simulink model "ev_pilot_handshake"  (R2024b)
settings: Solver=FixedStepAuto  StartTime=0.0  StopTime=5  FixedStep=1e-6  RelTol=1e-3
libraries: fl_lib x23, nesl_utility x13, ee_lib x2, simulink x1
settings Model: Creator=Shakeb  LastModifiedBy=Shakeb

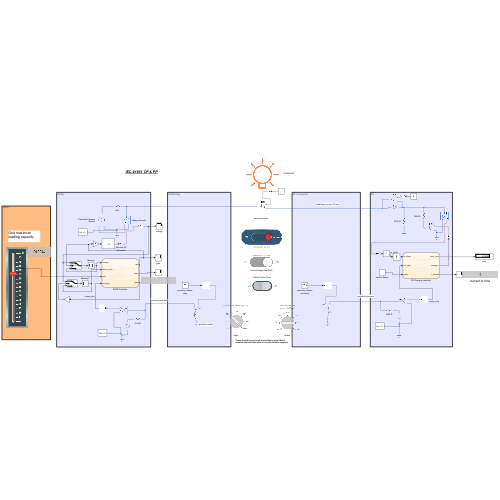
[thumbnail: Simulink's stored preview of the top-level diagram]
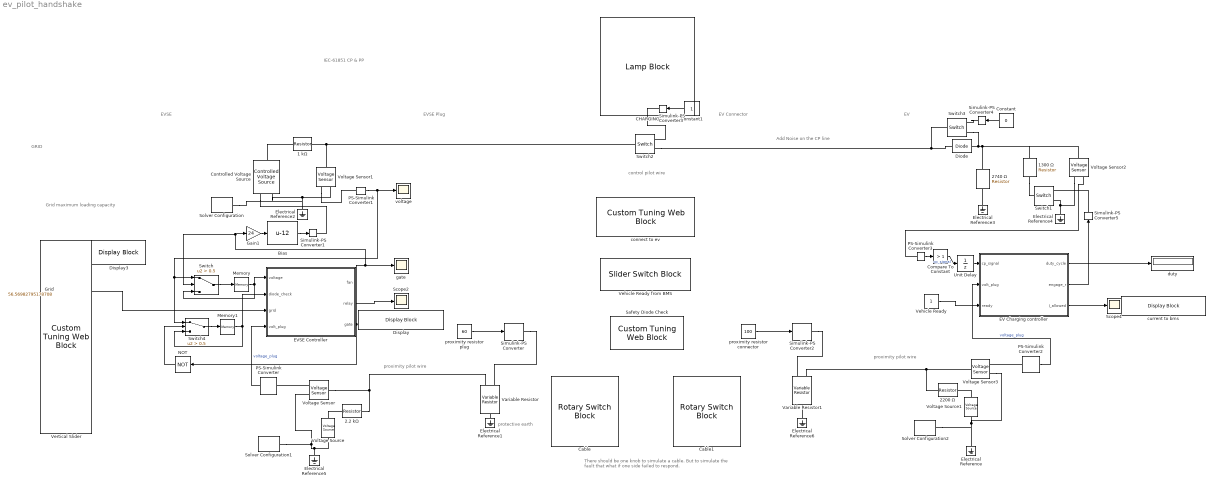
== system ev_pilot_handshake ==
  note: Grid maximum loading capacity
  note: GRID
  note: Add Noise on the CP line
  note: IEC-61851 CP & PP
  note: There should be one knob to simulate a cable. But to simulate the fault that what if one side failed to respond.
  note: protective earth
  note: control pilot wire
  note: proximity pilot wire
  note: EV
  note: EV Connector
  note: EVSE Plug
  note: EVSE
  note: proximity pilot wire
  1 kΩ : fl_lib/Electrical/Electrical Elements/Resistor  R=1000 Ohm  i_specify=off  i_priority=None  i=0 A  i_nominal_specify=off  i_nominal_value=1  i_nominal_unit=A  v_specify=off  v_priority=None  v=0 V  v_nominal_specify=off  v_nominal_value=1  v_nominal_unit=V
  1300 Ω : fl_lib/Electrical/Electrical Elements/Resistor  R=1300 Ohm  i_specify=off  i_priority=None  i=0 A  i_nominal_specify=off  i_nominal_value=1  i_nominal_unit=A  v_specify=off  v_priority=None  v=0 V  v_nominal_specify=off  v_nominal_value=1  v_nominal_unit=V
  2.2 kΩ : fl_lib/Electrical/Electrical Elements/Resistor  R=2200 Ohm  i_specify=off  i_priority=None  i=0 A  i_nominal_specify=off  i_nominal_value=1  i_nominal_unit=A  v_specify=off  v_priority=None  v=0 V  v_nominal_specify=off  v_nominal_value=1  v_nominal_unit=V
  2200 Ω : fl_lib/Electrical/Electrical Elements/Resistor  R=2200 Ohm  i_specify=off  i_priority=None  i=0 A  i_nominal_specify=off  i_nominal_value=1  i_nominal_unit=A  v_specify=off  v_priority=None  v=0 V  v_nominal_specify=off  v_nominal_value=1  v_nominal_unit=V
  2740 Ω : fl_lib/Electrical/Electrical Elements/Resistor  R=2740 Ohm  i_specify=off  i_priority=None  i=0 A  i_nominal_specify=off  i_nominal_value=1  i_nominal_unit=A  v_specify=off  v_priority=None  v=0 V  v_nominal_specify=off  v_nominal_value=1  v_nominal_unit=V
  Bias : Bias  Bias=-12  SaturateOnIntegerOverflow=off
  CHARGING : LampBlock  LabelPosition=Hide  Icon=LightingSwitch
  Cable : RotarySwitchBlock
      settings: Values={{'fault', '13A', '16A', '20A', '32A', '63A', 'short'}, [4500 1500 1000 680 220 100 60]}
  Cable1 : RotarySwitchBlock
      settings: Values={{'fault', '13A', '16A', '20A', '32A', '63A', 'short'}, [4500 1500 1000 680 220 100 60]}
  Compare To Constant : simulink/Logic and Bit Operations/Compare To Constant  relop=>  const=1  OutDataTypeStr=boolean
  Constant : Constant  Value=0
  Constant1 : Constant
  Controlled Voltage Source : fl_lib/Electrical/Electrical Sources/Controlled Voltage Source
  Diode : fl_lib/Electrical/Electrical Elements/Diode  Vf=0.6 V  Ron=0.3 Ohm  Goff=1e-8 1/Ohm  i_specify=off  i_priority=None  i=0 A  i_nominal_specify=off  i_nominal_value=1  i_nominal_unit=A  v_specify=off  v_priority=None  v=0 V  v_nominal_specify=off  v_nominal_value=1  v_nominal_unit=V
  Display : DisplayBlock  LabelPosition=Hide  Transparency=1
  Display3 : DisplayBlock  LabelPosition=Hide  Transparency=1
  EV Charging controller : Stateflow chart  TreatAsAtomicUnit=on
  EVSE Controller : Stateflow chart  TreatAsAtomicUnit=on
  Electrical Reference{,1..6} (7 alike) : fl_lib/Electrical/Electrical Elements/Electrical Reference
  Gain1 : Gain  Gain=24
  Grid : Constant  Value=56.56982795178708
  Memory : Memory  InitialCondition=12  InheritSampleTime=on
  Memory1 : Memory  InitialCondition=-12  InheritSampleTime=on
  NOT : Logic  Operator=NOT  IconShape=distinctive  AllPortsSameDT=off  OutDataTypeStr=boolean
  PS-Simulink Converter{,1..3} (4 alike) : nesl_utility/PS-Simulink Converter  PhysicalDomain=network_engine_domain  SubClassName=ps_output  LeftPortType=input  RightPortType=output  PseudoPeriodic=off  Frequencies=[]  VectorFormat=inherit  Unit=inherit  AffineConversion=off
  Safety Diode Check : CustomTuningWebBlock  LabelPosition=Hide  ShowInitialText=on  Configuration="{\"components\":[{\"name\":\"CustomSwitchStateComponent\",\"settings\":{\"position\":[0,0,1,1],\"states\":[{\"HitRegion\":{\"position\":[0,0,0.5,1]},\"Image\":{\"position\":[0.13,0,1,0.75],\"size\":[1,0.75],\"src\":\"data:image\\/svg+xml;base64,PHN2ZyB4bWxucz0iaHR0cDovL3d3dy53My5vcmcvMjAwMC9zdmciIHhtbG5zOnhsaW5rPSJodHRwOi8vd3d3LnczLm9yZy8xOTk5L3hsaW5rIiB2aWV3Qm94PSIwIDAgNzUgMjQuOCI+PGRlZnM+PHN0eWxlPi5jbHMtMXtmaWxsOnVybCgjcmFkaWFsLWdyYWRpZW50KTt9LmNscy0ye2ZpbGw6dXJsKCNyYWRpYWwtZ3JhZGllbnQtMik7fS5jbHMtM3tzdHJva2U6I2IyMDAwMDtzdHJva2Utd2lkdGg6MC4yNXB4O2ZpbGw6dXJsKCNsaW5lYXItZ3JhZGllbnQpO30uY2xzLTR7ZmlsbDp1cmwoI2xpbmVhci1ncmFkaWVudC0yKTt9LmNs ...(+3576 chars)\",\"srcOrientation\":\"Right\"},\"Label\":{\"color\":[0.5019607843137255,0.5019607843137255,0.5019607843137255],\"icon\":{\"size\":[0,0],\"src\":[],\"srcOrientation\":\"Right\"},\"iconOffset\":0,\"iconPlacement\":\"left\",\"opacity\":1,\"position\":[0.5,0.08],\"show\":true,\"text\":{\"content\":\"On\",\"font\":\"Helvetica\"}},\"Value\":0},{\"HitRegion\":{\"position\":[0,0.5,0.5,1]},\"Image\":{\"position\":[0.13,0,1,0.75],\"size\":[1,0.75],\"src\":\"data:image\\/svg+xml;base64,PHN2ZyB4bWxucz0iaHR0cDovL3d3dy53My5vcmcvMjAwMC9zdmciIHhtbG5zOnhsaW5rPSJodHRwOi8vd3d3LnczLm9yZy8xOTk5L3hsaW5rIiB2aWV3Qm94PSIwIDAgNzUgMjQuOCI+PGRlZnM+PHN0eWxlPi5jbHMtMXtmaWxsOnVybCgjcmFkaWFsLWdyYWRpZW50KTt9LmNscy0ye2ZpbGw6dXJsKCNyYWRpYWwtZ3JhZGllbnQtMik7fS5jbHMtM3tzdHJva2U6I2IyMDAwMDtzdHJva2Utd2lkdGg6MC4yNXB4O2ZpbGw6dXJsKCNsaW5lYXItZ3JhZGllbnQpO30uY2xzLTR7ZmlsbDp1cmwoI2xpbmVhci1ncmFkaWVudC0yKTt9LmNs ...(+3520 chars)\",\"srcOrientation\":\"Right\"},\"Label\":{\"color\":[0.5019607843137255,0.5019607843137255,0.5019607843137255],\"icon\":{\"size\":[0,0],\"src\":[],\"srcOrientation\":\"Right\"},\"iconOffset\":0,\"iconPlacement\":\"left\",\"opacity\":1,\"position\":[0.5,0.92],\"show\":true,\"text\":{\"content\":\"Off\",\"font\":\"Helvetica\"}},\"Value\":1}]}},{\"name\":\"BackgroundImageComponent\",\"settings\":{\"image\":{\"size\":[155,70],\"src\":\"default\",\"srcOrientation\":\"Right\"},\"position\":[0,0,1,1],\"scaleMode\":\"0\"}},{\"name\":\"ForegroundImageComponent\",\"settings\":{\"image\":{\"size\":[0,0],\"src\":\"default\",\"srcOrientation\":[]},\"isForeground\":1,\"position\":[0,0,1,1],\"scaleMode\":\"0\"}}],\"settings\":{\"BindingType\":\"param\",\"backgroundColor\":[0,0,255,\"1\"],\"backgroundOffset\":0.14,\"fixedAspectRatio\":\"on\",\"foregroundColor\":[234,234,234],\"showBackgroundColor\":false,\"variant\":\"rocker\",\"version\":\"R2024b\"},\"type\":\"Switch\"}"  CustomBackgroundColor="{\"color\":[1,1,1],\"show\":true}"
  Scope2 : Scope
  Scope4 : Scope
  Simulink-PS Converter{,1..5} (6 alike) : nesl_utility/Simulink-PS Converter  PhysicalDomain=network_engine_domain  SubClassName=ps_input  LeftPortType=input  RightPortType=output  PseudoPeriodic=off  Frequencies=[]  NoiseDistribution=none  NoiseParameters=[]  Unit=1  AffineConversion=off  FilteringAndDerivatives=provide  SimscapeFilterOrder=1  InputFilterTimeConstant=0.001  UdotUserProvided=0
  Solver Configuration : nesl_utility/Solver Configuration  PhysicalDomain=network_engine_domain  SubClassName=solver  LeftPortType=input  RightPortType=generic  Tones=[]  Harmonics=[]  SimulateNoise=off  Profile=off  UseLocalSampling=off  EnableSwitchedLinearOptims=on  FrequencyDomain=off  UseCCode=off  RelTol=0.001  AbsTol=0.001  MinStep=1e-09  ToWorkspace=off  RevertToSquareIcSolve=off  NumHomotopyIterations=100  PhasorMode=off  PhasorModeNumHarmonics=1  ConsistencySolver=NEWTON_XTOL_AFTER_FTOL  IndexReductionMethod=DerivativeReplacement  DoDC=off  ResidualTolerance=1e-09  ConsistencyTolSource=GLOBAL  ConsistencyAbsTol=0.001  ConsistencyRelTol=0.001  ConsistencyTolFactor=0.001  UseLocalSolver=off  LocalSolverChoice=NE_BACKWARD_EULER_ADVANCER  ResolveIndetEquations=on  FunctionEvalNumThread=1  LocalSolverSampleTime=0.001  DoFixedCost=off  MaxNonlinIter=3  MaxModeIter=2  ComputeImpulses=off  ImpulseIterations=2  LinearAlgebra=auto  LinearAlgebraNumThread=0  EquationFormulation=NE_TIME_EF  DelaysMemoryBudget=1024  AutomaticFiltering=on  FilteringTimeConstant=0.001  PartitionStorageMethod=AS_NEEDED  PartitionMemoryBudget=1024  PartitionMethod=ROBUST  MultibodyUseLocalSolver=off  MultibodyLocalSolverChoice=ODE1  MultibodyLocalSolverSampleTime=0.001
  Solver Configuration1 : nesl_utility/Solver Configuration  PhysicalDomain=network_engine_domain  SubClassName=solver  LeftPortType=input  RightPortType=generic  Tones=[]  Harmonics=[]  SimulateNoise=off  Profile=off  UseLocalSampling=off  EnableSwitchedLinearOptims=on  FrequencyDomain=off  UseCCode=off  RelTol=0.001  AbsTol=0.001  MinStep=1e-09  ToWorkspace=off  RevertToSquareIcSolve=off  NumHomotopyIterations=100  PhasorMode=off  PhasorModeNumHarmonics=1  ConsistencySolver=NEWTON_XTOL_AFTER_FTOL  IndexReductionMethod=DerivativeReplacement  DoDC=off  ResidualTolerance=1e-09  ConsistencyTolSource=GLOBAL  ConsistencyAbsTol=0.001  ConsistencyRelTol=0.001  ConsistencyTolFactor=0.001  UseLocalSolver=off  LocalSolverChoice=NE_BACKWARD_EULER_ADVANCER  ResolveIndetEquations=on  FunctionEvalNumThread=1  LocalSolverSampleTime=0.001  DoFixedCost=off  MaxNonlinIter=3  MaxModeIter=2  ComputeImpulses=off  ImpulseIterations=2  LinearAlgebra=auto  LinearAlgebraNumThread=0  EquationFormulation=NE_TIME_EF  DelaysMemoryBudget=1024  AutomaticFiltering=on  FilteringTimeConstant=0.001  PartitionStorageMethod=AS_NEEDED  PartitionMemoryBudget=1024  PartitionMethod=ROBUST  MultibodyUseLocalSolver=off  MultibodyLocalSolverChoice=ODE1  MultibodyLocalSolverSampleTime=0.001
  Solver Configuration2 : nesl_utility/Solver Configuration  PhysicalDomain=network_engine_domain  SubClassName=solver  LeftPortType=input  RightPortType=generic  Tones=[]  Harmonics=[]  SimulateNoise=off  Profile=off  UseLocalSampling=off  EnableSwitchedLinearOptims=on  FrequencyDomain=off  UseCCode=off  RelTol=0.001  AbsTol=0.001  MinStep=1e-09  ToWorkspace=off  RevertToSquareIcSolve=off  NumHomotopyIterations=100  PhasorMode=off  PhasorModeNumHarmonics=1  ConsistencySolver=NEWTON_XTOL_AFTER_FTOL  IndexReductionMethod=DerivativeReplacement  DoDC=off  ResidualTolerance=1e-09  ConsistencyTolSource=GLOBAL  ConsistencyAbsTol=0.001  ConsistencyRelTol=0.001  ConsistencyTolFactor=0.001  UseLocalSolver=off  LocalSolverChoice=NE_BACKWARD_EULER_ADVANCER  ResolveIndetEquations=on  FunctionEvalNumThread=1  LocalSolverSampleTime=0.001  DoFixedCost=off  MaxNonlinIter=3  MaxModeIter=2  ComputeImpulses=off  ImpulseIterations=2  LinearAlgebra=auto  LinearAlgebraNumThread=0  EquationFormulation=NE_TIME_EF  DelaysMemoryBudget=1024  AutomaticFiltering=on  FilteringTimeConstant=0.001  PartitionStorageMethod=AS_NEEDED  PartitionMemoryBudget=1024  PartitionMethod=ROBUST  MultibodyUseLocalSolver=off  MultibodyLocalSolverChoice=ODE1  MultibodyLocalSolverSampleTime=0.001
  Switch : Switch  Criteria=u2 > Threshold  Threshold=0.5  SaturateOnIntegerOverflow=off  InputSameDT=off
  Switch1 : fl_lib/Electrical/Electrical Elements/Switch  R_closed=0.01 Ohm  G_open=1e-8 1/Ohm  Threshold=0.5  i_specify=off  i_priority=None  i=0 A  i_nominal_specify=off  i_nominal_value=1  i_nominal_unit=A  v_specify=off  v_priority=None  v=0 V  v_nominal_specify=off  v_nominal_value=1  v_nominal_unit=V
  Switch2 : fl_lib/Electrical/Electrical Elements/Switch  R_closed=0.001 Ohm  G_open=1e-8 1/Ohm  Threshold=0.5  i_specify=off  i_priority=None  i=0 A  i_nominal_specify=off  i_nominal_value=1  i_nominal_unit=A  v_specify=off  v_priority=None  v=0 V  v_nominal_specify=off  v_nominal_value=1  v_nominal_unit=V
  Switch3 : fl_lib/Electrical/Electrical Elements/Switch  R_closed=0.001 Ohm  G_open=1e-8 1/Ohm  Threshold=0.5  i_specify=off  i_priority=None  i=0 A  i_nominal_specify=off  i_nominal_value=1  i_nominal_unit=A  v_specify=off  v_priority=None  v=0 V  v_nominal_specify=off  v_nominal_value=1  v_nominal_unit=V
  Switch4 : Switch  Criteria=u2 > Threshold  Threshold=0.5  SaturateOnIntegerOverflow=off  InputSameDT=off
  Unit Delay : UnitDelay  InitialCondition=1  SampleTime=-1  HasFrameUpgradeWarning=on
  Variable Resistor : fl_lib/Electrical/Electrical Elements/Variable Resistor  Rmin=0 Ohm  thermalEnable=false  thermal_mass=1 J/K  i_specify=off  i_priority=None  i=0 A  i_nominal_specify=off  i_nominal_value=1  i_nominal_unit=A  v_specify=off  v_priority=None  v=0 V  v_nominal_specify=off  v_nominal_value=1  v_nominal_unit=V  T_specify=off  T_priority=None  T=300 K  T_nominal_specify=off  T_nominal_value=1  T_nominal_unit=K
  Variable Resistor1 : fl_lib/Electrical/Electrical Elements/Variable Resistor  Rmin=0 Ohm  thermalEnable=false  thermal_mass=1 J/K  i_specify=off  i_priority=None  i=0 A  i_nominal_specify=off  i_nominal_value=1  i_nominal_unit=A  v_specify=off  v_priority=None  v=0 V  v_nominal_specify=off  v_nominal_value=1  v_nominal_unit=V  T_specify=off  T_priority=None  T=300 K  T_nominal_specify=off  T_nominal_value=1  T_nominal_unit=K
  Vehicle Ready : Constant
  Vehicle Ready from BMS : SliderSwitchBlock
      settings: Values={{'Off', 'On'}, [0 1]}
  Vertical Slider : CustomTuningWebBlock  LabelPosition=Hide  ShowInitialText=on  Configuration="{\"components\":[{\"name\":\"LinearScaleComponent\",\"settings\":{\"bounds\":{\"max\":80,\"min\":0,\"tickInterval\":\"auto\"},\"internalTickHeightScaleFactor\":0.5,\"labelColor\":[255,255,200],\"labelFont\":{\"font\":\"Arial\",\"fontSize\":12},\"labelOffset\":0.05,\"labelTransparency\":1,\"needleImage\":{\"size\":[596,842],\"src\":\"data:image\\/svg+xml;base64,PD94bWwgdmVyc2lvbj0iMS4wIiBlbmNvZGluZz0idXRmLTgiPz4NCjwhLS0gR2VuZXJhdG9yOiBBZG9iZSBJbGx1c3RyYXRvciAyNS4wLjAsIFNWRyBFeHBvcnQgUGx1Zy1JbiAuIFNWRyBWZXJzaW9uOiA2LjAwIEJ1aWxkIDApICAtLT4NCjxzdmcgdmVyc2lvbj0iMS4xIg0KCSBpZD0ic3ZnOCIgeG1sbnM6Y2M9Imh0dHA6Ly9jcmVhdGl2ZWNvbW1vbnMub3JnL25zIyIgeG1sbnM6ZGM9Imh0dHA6Ly9wdXJsLm9yZy9kYy9lbGVtZW50cy8xLjEvIiB4bWxuczppbmtzY2FwZT0iaHR0cDovL3d3dy5pbmtzY2FwZS5vcmcvbmFtZXNw ...(+2420 chars)\",\"srcOrientation\":\"horizontal\"},\"needleOffset\":[0.0642123287671233,-0.8044596912521441],\"needleSize\":{\"height\":0.07668067226890757,\"width\":0.4337797619047619},\"position\":[0.03623949579831933,0.2829861111111111,0.6088789682539683,0.9196428571428571],\"referencePoint\":\"auto\",\"scaleColors\":[],\"scaleColorsSize\":0.2,\"scaleDirection\":\"BT\",\"showLabels\":1,\"showMinorTicks\":0,\"showSpanLine\":1,\"showTicks\":1,\"tickColor\":[252,252,197],\"tickTransparency\":1,\"valueBarColor\":[0,114,189],\"valueBarOffset\":-0.27,\"valueBarSize\":0.1,\"valueBarTransparency\":1}},{\"name\":\"BackgroundImageComponent\",\"settings\":{\"image\":{\"size\":[380,101],\"src\":\"data:image\\/svg+xml;base64,PHN2ZyB4bWxucz0iaHR0cDovL3d3dy53My5vcmcvMjAwMC9zdmciIHhtbG5zOnhsaW5rPSJodHRwOi8vd3d3LnczLm9yZy8xOTk5L3hsaW5rIiB2aWV3Qm94PSIwIDAgMzgwIDEwMSI+PGRlZnM+PHN0eWxlPi5jbHMtMXtmaWxsOiMwMDJiNDI7fS5jbHMtMntmaWxsOiM0MjcwODI7fS5jbHMtM3tmaWxsOnVybCgjcmFkaWFsLWdyYWRpZW50KTt9LmNscy00e2ZpbGw6I2M4YzhjODtzdHJva2U6IzAwMDt9PC9zdHlsZT48cmFkaWFsR3JhZGllbnQgaWQ9InJhZGlhbC1ncmFkaWVudCIgY3g9IjE5MCIgY3k9IjUwLjUiIHI9IjI2OS4yMSIgZ3JhZGllbnRVbml0cz0idXNlclNwYWNlT25Vc2UiPjxzdG9wIG9mZnNldD0iMC4wMSIgc3RvcC1jb2xvcj0iIzNlNGY1OCIvPjxzdG9wIG9mZnNldD0iMC4wNiIgc3RvcC1jb2xvcj0iIzQ0NTc2MSIvPjxzdG9wIG9mZnNldD0iMC4xNSIgc3RvcC1jb2xvcj0iIzU1NmE3NiIvPjxzdG9wIG9mZnNldD0iMC4yNSIgc3RvcC1jb2xvcj0iIzZkODg5NSIvPjxzdG9wIG9mZnNldD0iMC4zOCIgc3RvcC1jb2xvcj0iIzhmYjJjMyIvPjxzdG9wIG9mZnNldD0iMC41MiIgc3RvcC1jb2xvcj0iI2I2ZTRmYSIvPjxzdG9wIG9mZnNldD0iMSIgc3RvcC1jb2xvcj0iIzE1NDY1NyIvPjwvcmFkaWFsR3JhZGllbnQ+PC9kZWZzPjxnIGlkPSJmcmFtZSI+PGcgaWQ9IkxheWVyXzIiIGRhdGEtbmFtZT0iTGF5ZXIgMiI+PGcgaWQ9IkxheWVyXzEtMiIgZGF0YS1uYW1lPSJMYXllciAxLTIiPjxyZWN0IGlkPSJyZWN0MTAzNiIgY2xhc3M9ImNscy0xIiB4PSIxMSIgeT0iMTEiIHdpZHRoPSIzNTgiIGhlaWdodD0iNzkiLz48cGF0aCBpZD0icGF0aDEwMzgiIGNsYXNzPSJjbHMtMiIgZD0iTTgsOFY5M0gzNzJWOFpNMzY5LDkwSDExVjExSDM2OVoiLz48cGF0aCBpZD0icGF0aDEwNDAiIGNsYXNzPSJjbHMtMyIgZD0iTTAsMFYxMDFIMzgwVjBaTTM3Miw5M0g4VjhIMzcyWiIvPjwvZz48L2c+PC9nPjxnIGlkPSJ0cmFjayI+PHBhdGggaWQ9InJlY3QxNjExIiBjbGFzcz0iY2xzLTQiIGQ9Ik0zMy4zNywyNi41OUgzNDYuNjNjNCwwLDcuMjUsMi42LDcuMjUsNS44MWgwYzAsMy4yMS0zLjI1LDUuODItNy4yNSw1LjgySDMzLjM3Yy00LDAtNy4yNS0yLjYxLTcuMjUtNS44MmgwQzI2LjEyLDI5LjE5LDI5LjM3LDI2LjU5LDMzLjM3LDI2LjU5WiIvPjwvZz48L3N2Zz4=\",\"srcOrientation\":\"horizontal\"},\"position\":[0,0,1,1],\"scaleMode\":\"0\"}},{\"name\":\"ForegroundImageComponent\",\"settings\":{\"image\":{\"size\":[0,0],\"src\":\"default\",\"srcOrientation\":[]},\"isForeground\":1,\"position\":[0,0,1,1],\"scaleMode\":\"0\"}}],\"settings\":{\"BindingType\":\"param\",\"aspectRatio\":3.7777777777777777,\"backgroundColor\":[0,0,0,\"1\"],\"backgroundOffset\":0,\"backgroundOpacity\":1,\"fixedAspectRatio\":\"on\",\"foregroundColor\":[252,252,196],\"orientation\":\"vertical\",\"showBackgroundColor\":false,\"value\":0,\"version\":\"R2023a\"},\"type\":\"LinearGauge\"}"
  Voltage Sensor{,1..3} (4 alike) : fl_lib/Electrical/Electrical Sensors/Voltage Sensor
  Voltage Source : ee_lib/Sources/Voltage Source  dc_voltage=5 V  ac_voltage=0 V  ac_shift=0 rad  ac_frequency=60 Hz  noise_mode=ee.enum.sources.noise.Disabled  PSD=0 V^2/Hz  sample_time=1e-3 s  repeatability=ee.enum.sources.repeatability.NotRepeatable  user_seed=0  auto_seed=3890346746  i_specify=off  i_priority=None  i=0 A  i_nominal_specify=off  i_nominal_value=1  i_nominal_unit=A  v_specify=off  v_priority=None  v=0 V  v_nominal_specify=off  v_nominal_value=1  v_nominal_unit=V
  Voltage Source1 : ee_lib/Sources/Voltage Source  dc_voltage=5 V  ac_voltage=0 V  ac_shift=0 rad  ac_frequency=60 Hz  noise_mode=ee.enum.sources.noise.Disabled  PSD=0 V^2/Hz  sample_time=1e-3 s  repeatability=ee.enum.sources.repeatability.NotRepeatable  user_seed=0  auto_seed=3499211588  i_specify=off  i_priority=None  i=0 A  i_nominal_specify=off  i_nominal_value=1  i_nominal_unit=A  v_specify=off  v_priority=None  v=0 V  v_nominal_specify=off  v_nominal_value=1  v_nominal_unit=V
  connect to ev : CustomTuningWebBlock  LabelPosition=Hide  ShowInitialText=on  Configuration="{\"components\":[{\"name\":\"CustomSwitchStateComponent\",\"settings\":{\"position\":[0,0,1,1],\"states\":[{\"HitRegion\":{\"position\":[0,0,0.5,1]},\"Image\":{\"position\":[0,0,1,1],\"size\":[1,1],\"src\":\"data:image\\/svg+xml;base64,PD94bWwgdmVyc2lvbj0iMS4wIiBlbmNvZGluZz0idXRmLTgiPz4NCjwhLS0gR2VuZXJhdG9yOiBBZG9iZSBJbGx1c3RyYXRvciAyNS4yLjEsIFNWRyBFeHBvcnQgUGx1Zy1JbiAuIFNWRyBWZXJzaW9uOiA2LjAwIEJ1aWxkIDApICAtLT4NCjxzdmcgdmVyc2lvbj0iMS4xIiB4bWxucz0iaHR0cDovL3d3dy53My5vcmcvMjAwMC9zdmciIHhtbG5zOnhsaW5rPSJodHRwOi8vd3d3LnczLm9yZy8xOTk5L3hsaW5rIiB4PSIwcHgiIHk9IjBweCINCgkgdmlld0JveD0iMCAwIDc2IDI5IiBzdHlsZT0iZW5hYmxlLWJhY2tncm91bmQ6bmV3 ...(+5404 chars)\",\"srcOrientation\":\"Right\"},\"Label\":{\"color\":[0.9882352941176471,0.9882352941176471,0.7725490196078432],\"icon\":{\"size\":[0,0],\"src\":[],\"srcOrientation\":\"Right\"},\"iconOffset\":0,\"iconPlacement\":\"left\",\"opacity\":1,\"position\":[0.5,0.14],\"show\":true,\"text\":{\"content\":\"Off\",\"font\":\"Helvetica\"}},\"Value\":0},{\"HitRegion\":{\"position\":[0,0.5,0.5,1]},\"Image\":{\"position\":[0,0,1,1],\"size\":[1,1],\"src\":\"data:image\\/svg+xml;base64,PD94bWwgdmVyc2lvbj0iMS4wIiBlbmNvZGluZz0idXRmLTgiPz4NCjwhLS0gR2VuZXJhdG9yOiBBZG9iZSBJbGx1c3RyYXRvciAyNS4yLjEsIFNWRyBFeHBvcnQgUGx1Zy1JbiAuIFNWRyBWZXJzaW9uOiA2LjAwIEJ1aWxkIDApICAtLT4NCjxzdmcgdmVyc2lvbj0iMS4xIiB4bWxucz0iaHR0cDovL3d3dy53My5vcmcvMjAwMC9zdmciIHhtbG5zOnhsaW5rPSJodHRwOi8vd3d3LnczLm9yZy8xOTk5L3hsaW5rIiB4PSIwcHgiIHk9IjBweCINCgkgdmlld0JveD0iMCAwIDc2IDI5IiBzdHlsZT0iZW5hYmxlLWJhY2tncm91bmQ6bmV3 ...(+5404 chars)\",\"srcOrientation\":\"Right\"},\"Label\":{\"color\":[0.9882352941176471,0.9882352941176471,0.7725490196078432],\"icon\":{\"size\":[0,0],\"src\":[],\"srcOrientation\":\"Right\"},\"iconOffset\":0,\"iconPlacement\":\"left\",\"opacity\":1,\"position\":[0.5,0.86],\"show\":true,\"text\":{\"content\":\"Connect\",\"font\":\"Helvetica\"}},\"Value\":1}]}},{\"name\":\"BackgroundImageComponent\",\"settings\":{\"image\":{\"size\":[140,55],\"src\":\"default\",\"srcOrientation\":\"Right\"},\"position\":[0,0,1,1],\"scaleMode\":\"0\"}},{\"name\":\"ForegroundImageComponent\",\"settings\":{\"image\":{\"size\":[0,0],\"src\":\"default\",\"srcOrientation\":[]},\"isForeground\":1,\"position\":[0,0,1,1],\"scaleMode\":\"0\"}}],\"settings\":{\"BindingType\":\"param\",\"backgroundColor\":[0,0,255,\"1\"],\"backgroundOffset\":0.14,\"fixedAspectRatio\":\"on\",\"foregroundColor\":[234,234,234],\"showBackgroundColor\":false,\"variant\":\"slider\",\"version\":\"R2024b\"},\"type\":\"Switch\"}"
  current to bms : DisplayBlock  LabelPosition=Hide  Transparency=1
  duty : Display
  gate : Scope
  proximity resistor connector : Constant  Value=100
  proximity resistor plug : Constant  Value=60
  voltage : Scope
  wires:
  proximity resistor plug/1 -> Simulink-PS Converter/1
  PS-Simulink Converter/1 -> EVSE Controller/4(volt_plug)  "voltage_plug"
  Gain1/1 -> Bias/1
  Bias/1 -> Simulink-PS Converter1/1
  EVSE Controller/3(gate) -> Gain1/1, Switch/2, gate/1, NOT/1
  proximity resistor connector/1 -> Simulink-PS Converter2/1
  Constant1/1 -> Simulink-PS Converter3/1
  Switch/1 -> Memory/1
  Memory/1 -> Switch/3, EVSE Controller/1(voltage)
  Constant/1 -> Simulink-PS Converter4/1
  EVSE Controller/2(relay) -> Scope2/1
  PS-Simulink Converter1/1 -> Switch4/1, Switch/1, voltage/1
  Switch4/1 -> Memory1/1
  Memory1/1 -> Switch4/3, EVSE Controller/2(diode_check)
  NOT/1 -> Switch4/2
  PS-Simulink Converter3/1 -> Compare To Constant/1
  EV Charging controller/1(duty_cycle) -> duty/1
  PS-Simulink Converter2/1 -> EV Charging controller/2(volt_plug)  "voltage_plug"
  Vehicle Ready/1 -> EV Charging controller/3(ready)
  EV Charging controller/2(engage_r) -> Simulink-PS Converter5/1
  EV Charging controller/3(I_allowed) -> Scope4/1
  Compare To Constant/1 -> Unit Delay/1  "cp_signal"
  Unit Delay/1 -> EV Charging controller/1(cp_signal)
  Grid/1 -> EVSE Controller/3(grid)
  connections:
  Voltage Source/LConn1 -- 2.2 kΩ/LConn1
  Simulink-PS Converter/RConn1 -- Variable Resistor/LConn1
  2.2 kΩ/RConn1 -- Voltage Sensor/LConn1 -- Variable Resistor/LConn2
  Electrical Reference1/LConn1 -- Variable Resistor/RConn1
  Voltage Sensor/RConn1 -- PS-Simulink Converter/LConn1
  Controlled Voltage Source/RConn1 -- Simulink-PS Converter1/RConn1
  Controlled Voltage Source/LConn1 -- 1 kΩ/LConn1
  Voltage Sensor1/LConn1 -- 1 kΩ/RConn1 -- Switch2/LConn1
  Voltage Sensor1/RConn1 -- PS-Simulink Converter1/LConn1
  2740 Ω/LConn1 -- Voltage Sensor2/LConn1 -- 1300 Ω/LConn1 -- Switch3/RConn2 -- Diode/RConn1
  Electrical Reference3/LConn1 -- 2740 Ω/RConn1
  1300 Ω/RConn1 -- Switch1/LConn1
  Electrical Reference4/LConn1 -- Voltage Sensor2/RConn2 -- Switch1/RConn2
  Simulink-PS Converter2/RConn1 -- Variable Resistor1/LConn1
  Voltage Sensor3/LConn1 -- 2200 Ω/RConn1 -- Variable Resistor1/LConn2
  PS-Simulink Converter2/LConn1 -- Voltage Sensor3/RConn1
  Voltage Source1/LConn1 -- 2200 Ω/LConn1
  Electrical Reference6/LConn1 -- Variable Resistor1/RConn1
  Simulink-PS Converter3/RConn1 -- Switch2/RConn1
  Switch2/RConn2 -- Switch3/LConn1 -- Diode/LConn1
  Simulink-PS Converter4/RConn1 -- Switch3/RConn1
  PS-Simulink Converter3/LConn1 -- Voltage Sensor2/RConn1
  Voltage Sensor/RConn2 -- Solver Configuration1/RConn1 -- Voltage Source/RConn1 -- Electrical Reference5/LConn1
  Voltage Sensor3/RConn2 -- Electrical Reference/LConn1 -- Solver Configuration2/RConn1 -- Voltage Source1/RConn1
  Controlled Voltage Source/RConn2 -- Solver Configuration/RConn1 -- Electrical Reference2/LConn1 -- Voltage Sensor1/RConn2
  Simulink-PS Converter5/RConn1 -- Switch1/RConn1

== stateflow chart ev_pilot_handshake/EVSE Controller ==
  state Proximity [parallel]
    settings: executionOrder=1
    state short_ckt
      duty_p=0.025;
    state fault3
      duty_p=0.025;
    state A63
      duty_p=((63/2.5)+64)*0.01;
    state A32
      duty_p=(32/0.6)*0.01;
    state A20
      duty_p=(20/0.6)*0.01;
    state A16
      duty_p=(16/0.6)*0.01;
    state A13
      duty_p=(13/0.6)*0.01;
    (default) -> short_ckt
    A63 -> short_ckt [order 1] : [volt_plug<0.19]
    short_ckt -> A63 : [volt_plug>0.19]
    A13 -> fault3 [order 2] : [volt_plug>2.15]
    fault3 -> A13 : [volt_plug<2.15]
    A63 -> A32 [order 2] : [volt_plug>0.35]
    A32 -> A20 [order 2] : [volt_plug>1.05]
    A20 -> A16 [order 2] : [volt_plug>1.45]
    A16 -> A13 [order 2] : [volt_plug>1.95]
    A20 -> A32 [order 1] : [volt_plug<0.6]
    A16 -> A20 [order 1] : [volt_plug<1.25]
    A13 -> A16 [order 1] : [volt_plug<1.65]
    A32 -> A63 [order 1] : [volt_plug<0.35]
  state Grid_health [parallel]
    settings: executionOrder=2
    state not_allowed
      duty_g=0.025;
    state allowed_6_51
      duty_g = (grid/0.6)*0.01;
    state allowed_52_80
      duty_g = ((grid/2.5)+64)*0.01
    (default) -> not_allowed
    not_allowed -> allowed_6_51 : [grid>=6]
    allowed_6_51 -> allowed_52_80 [order 2] : [grid>51]
    allowed_6_51 -> not_allowed [order 1] : [grid<6]
    allowed_52_80 -> allowed_6_51 : [grid<50]
  state Control [parallel]
    duty_i = min(duty_p,duty_g)
    settings: executionOrder=3
    state NotConnected
      gate=1;
      relay=0;
    state Connected
      relay=0;
      state high
        gate=1;
      state low
        gate=0;
      Control.Connected.high -> Control.Connected.low : [after(0.001 * duty_i, sec)]
      (default) -> Control.Connected.high
      Control.Connected.low -> Control.Connected.high : [after(0.001 * (1-duty_i), sec)]
    state Charging_ventilation
      entry:
      fan=0;
      relay=0;
      during:
      relay=1;
      fan=1;
      exit:
      fan=0;
      relay=0;
      state low
        gate=0;
      state high
        gate=1;
      Control.Charging_ventilation.high -> Control.Charging_ventilation.low : [after(0.001 * duty_i, sec)]
      (default) -> Control.Charging_ventilation.high
      Control.Charging_ventilation.low -> Control.Charging_ventilation.high : [after(0.001 * (1-duty_i), sec)]
    state Charging
      entry:
      relay=0;
      during:
      relay=1;
      exit:
      relay=0;
      state high
        gate=1;
      state low
        gate=0;
      Control.Charging.high -> Control.Charging.low [order 3] : [after(0.001 * duty_i, sec)]
      Control.Charging.low -> Control.Charging.high : [after(0.001 * (1-duty_i), sec)]
    state fault
      relay=0;
      state EVSE_fail
      state CP_ground
      CP_ground -> EVSE_fail [order 2] : [voltage<0]
      EVSE_fail -> CP_ground : [voltage>0]
    (default) -> NotConnected
    NotConnected -> Connected : [voltage<10]
    Connected -> NotConnected [order 1] : [voltage>10]
    Control.Charging.high -> Connected [order 1] : [voltage>7]{relay=0;}
    Connected -> Control.Charging.high [order 2] : [voltage<7]
    Charging_ventilation -> Control.Charging.high [order 1] : [voltage>5]
    Control.Charging.high -> Charging_ventilation [order 2] : [voltage<4]
    Charging_ventilation -> CP_ground [order 2] : [voltage<2]
    CP_ground -> Charging_ventilation [order 1] : [voltage>2]
  state Safety [parallel]
    settings: executionOrder=4
    state okay
    state fault
      relay=0;
      gate=1;
    (default) -> okay
    okay -> Safety.fault : [gate == 0 && diode_check > -10]
  data: fan output; relay output; voltage input; diode_check input; grid input; volt_plug input; duty_i local; gate output =1; duty_g local =0.025; duty_p local =0.025

== stateflow chart ev_pilot_handshake/EV Charging controller ==
  state Proximity [parallel]
    settings: executionOrder=1
    state short_ckt
      duty_i=0.025;
    state fault3
      duty_i=0.025;
    state A63
      duty_i=((63/2.5)+64)*0.01;
    state A32
      duty_i=(32/0.6)*0.01;
    state A20
      duty_i=(20/0.6)*0.01;
    state A16
      duty_i=(16/0.6)*0.01;
    state A13
      duty_i=(13/0.6)*0.01;
    (default) -> short_ckt
    A63 -> short_ckt [order 1] : [volt_plug<0.19]
    short_ckt -> A63 : [volt_plug>0.19]
    A13 -> fault3 [order 2] : [volt_plug>2.15]
    fault3 -> A13 : [volt_plug<2.15]
    A63 -> A32 [order 2] : [volt_plug>0.35]
    A32 -> A20 [order 2] : [volt_plug>1.05]
    A20 -> A16 [order 2] : [volt_plug>1.45]
    A16 -> A13 [order 2] : [volt_plug>1.95]
    A20 -> A32 [order 1] : [volt_plug<0.6]
    A16 -> A20 [order 1] : [volt_plug<1.25]
    A13 -> A16 [order 1] : [volt_plug<1.65]
    A32 -> A63 [order 1] : [volt_plug<0.35]
  state Duty_calculate [parallel]
    settings: executionOrder=2
    state pulse_high
      entry:
      t_high=0;
      during:
      t_high = t_high+1;
    state pulse_low
      entry:
      t_low=0;
      during:
      t_low = t_low+1;
    (default) -> pulse_high
    pulse_high -> pulse_low : [cp_signal == 0]
    pulse_low -> pulse_high : [cp_signal == 1]{duty_cycle=(t_high/(t_high+t_low));
        | duty_accepted = min(duty_cycle, duty_i);}
  state Current_calculation [parallel]
    settings: executionOrder=3
    state NA
      I_allowed=0;
    state A6
      I_allowed=6;
    state normal
      I_allowed=duty_accepted*0.6*100;
    state ver_big
      I_allowed=80;
    state Na
      I_allowed=0;
    state big
      I_allowed=((duty_accepted*100) - 64)*2.5;
    (default) -> NA
    NA -> A6 : [duty_accepted>=0.08]
    A6 -> normal [order 2] : [duty_accepted>=0.10 ]
    A6 -> NA [order 1] : [duty_accepted<0.08]
    normal -> A6 [order 1] : [duty_accepted<0.1]
    normal -> big [order 2] : [duty_accepted>=0.85 ]
    big -> normal [order 1] : [duty_accepted<0.85]
    ver_big -> Na [order 2] : [duty_accepted>=0.97 ]
    big -> ver_big [order 2] : [duty_accepted>=0.96]
    Na -> ver_big : [duty_accepted<0.97]
    ver_big -> big [order 1] : [duty_accepted<0.96]
  state Charging_logic [parallel]
    settings: executionOrder=4
    state not_charging
      engage_r=0;
    state charging
      engage_r=1;
    (default) -> not_charging
    not_charging -> charging : [I_allowed>=6 && ready==1]
    charging -> not_charging : [after(0.001, sec) && (I_allowed < 6 || ready ~= 1)]
  data: cp_signal input; volt_plug input; duty_cycle output; t_high local; t_low local; duty_i local; engage_r output =0; I_allowed output; ready input; duty_accepted local =0
